simulink subsystem "variantGrad"  (R2023a)
settings: Solver=VariableStepAuto  StartTime=0.0  StopTime=10.0  RelTol=1e-3
settings Model: Creator=KozlovM  LastModifiedBy=motya

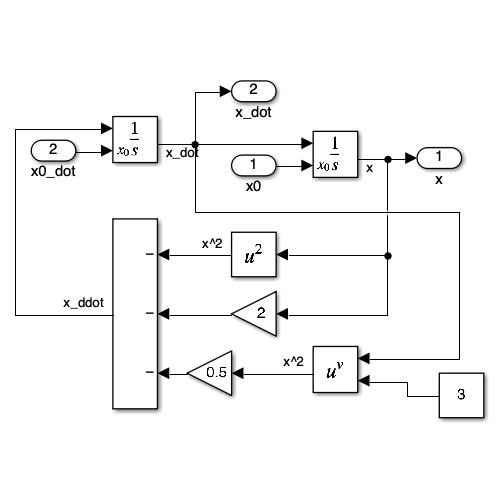
[thumbnail: Simulink's stored preview of the top-level diagram]
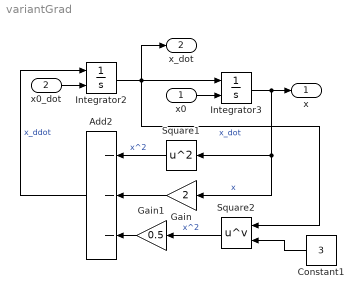
== system variantGrad ==
  x0 : Inport
  x0_dot : Inport  Port=2
  Add2 : Sum  Inputs=---
  Constant1 : Constant  Value=3
  Gain : Gain  Gain=2
  Gain1 : Gain  Gain=0.5
  Integrator2 : Integrator  InitialConditionSource=external
  Integrator3 : Integrator  InitialConditionSource=external  InitialCondition=2
  Square1 : Math  Operator=square
  Square2 : Math  Operator=pow
  x : Outport
  x_dot : Outport  Port=2
  wires:
  Square1/1 -> Add2/1  "x^2"
  Gain/1 -> Add2/2
  Gain1/1 -> Add2/3
  Constant1/1 -> Square2/2
  Square2/1 -> Gain1/1  "x^2"
  x0_dot/1 -> Integrator2/2
  Add2/1 -> Integrator2/1  "x_ddot"
  x0/1 -> Integrator3/2
  Integrator2/1 -> x_dot/1, Integrator3/1, Square2/1  "x_dot"
  Integrator3/1 -> Gain/1, Square1/1, x/1  "x"
